simulink model "model_graphicSim_Circuit"  (R2022a)
settings: Solver=FixedStepAuto  StartTime=0.0  StopTime=inf  RelTol=1e-3
values from neighbouring files (symbols this model uses):
  A = 9    [A_circuit_V2_25000.mat]    (also in A_circuit_V2_3167.mat; A_circuit_V3_30000.mat; A_circuit_V3_60000.mat; Configuration.m)
  d = 699840    [A_circuit_V2_25000.mat]    (also in A_circuit_V2_3167.mat; A_circuit_V3_30000.mat; A_circuit_V3_60000.mat; Configuration.m)
  egoID = 1    [A_circuit_V2_25000.mat]    (also in A_circuit_V2_3167.mat; A_circuit_V3_30000.mat; A_circuit_V3_60000.mat; Configuration.m)
  frontDistCG = 3.7    [A_circuit_V2_25000.mat]    (also in A_circuit_V2_3167.mat; A_circuit_V3_30000.mat; A_circuit_V3_60000.mat; Configuration.m)
  gridvx = [-5 -4.72222222222 -4.44444444444 -4.16666666667 -3.88888888889 -3.61111111111 -3.33333333333 -3.05555555556 -2.77777777778 -2.5 0 0.277777777778 ... (70 elements, 10x7)]    [A_circuit_V2_25000.mat]    (also in A_circuit_V2_3167.mat; A_circuit_V3_30000.mat; A_circuit_V3_60000.mat; circuit_10000_P2.mat)
  gridvy = [-70 -68.4444444444 -66.8888888889 -65.3333333333 -63.7777777778 -62.2222222222 -60.6666666667 -59.1111111111 -57.5555555556 -56 -50 -48.4444444444 ... (70 elements, 10x7)]    [A_circuit_V2_25000.mat]    (also in A_circuit_V2_3167.mat; A_circuit_V3_30000.mat; A_circuit_V3_60000.mat; circuit_10000_P2.mat)
  gridx = [-85 -84.6666666667 -84.3333333333 -84 -83.6666666667 -83.3333333333 -83 -82.6666666667 -82.3333333333 -82 -55 -54.6666666667 ... (70 elements, 10x7)]    [A_circuit_V2_25000.mat]    (also in A_circuit_V2_3167.mat; A_circuit_V3_30000.mat; A_circuit_V3_60000.mat; circuit_10000_P2.mat)
  gridy = [-70 -69.3333333333 -68.6666666667 -68 -67.3333333333 -66.6666666667 -66 -65.3333333333 -64.6666666667 -64 -50 -49.3333333333 ... (70 elements, 10x7)]    [A_circuit_V2_25000.mat]    (also in A_circuit_V2_3167.mat; A_circuit_V3_30000.mat; A_circuit_V3_60000.mat; circuit_10000_P2.mat)
  gridyaw = [-504 -489.6 -475.2 -460.8 -446.4 -432 -417.6 -403.2 -388.8 -374.4 -360 -345.6 ... (70 elements, 10x7)]    [A_circuit_V2_25000.mat]    (also in A_circuit_V2_3167.mat; A_circuit_V3_30000.mat; A_circuit_V3_60000.mat; circuit_10000_P2.mat)
  lb_angSt = -1080    [A_circuit_V2_25000.mat]    (also in A_circuit_V2_3167.mat; A_circuit_V3_30000.mat; A_circuit_V3_60000.mat; Configuration.m = -900)
  lbvx = 0    [A_circuit_V2_25000.mat]    (also in A_circuit_V2_3167.mat; A_circuit_V3_30000.mat; A_circuit_V3_60000.mat; Configuration.m = -2)
  lbvy = -50    [A_circuit_V2_25000.mat]    (also in A_circuit_V2_3167.mat; A_circuit_V3_30000.mat; A_circuit_V3_60000.mat; Configuration.m = -20)
  lbx = -55    [A_circuit_V2_25000.mat]    (also in A_circuit_V2_3167.mat; A_circuit_V3_30000.mat; A_circuit_V3_60000.mat; Configuration.m = 0)
  lby = -50    [A_circuit_V2_25000.mat]    (also in A_circuit_V2_3167.mat; A_circuit_V3_30000.mat; A_circuit_V3_60000.mat; Configuration.m = 2)
  leftDistCG = 0.9    [A_circuit_V2_25000.mat]    (also in A_circuit_V2_3167.mat; A_circuit_V3_30000.mat; A_circuit_V3_60000.mat; Configuration.m)
  M = 5    [A_circuit_V2_25000.mat]    (also in A_circuit_V2_3167.mat; A_circuit_V3_30000.mat; A_circuit_V3_60000.mat; Configuration.m)
  N = 10    [A_circuit_V2_25000.mat]    (also in A_circuit_V2_3167.mat; A_circuit_V3_30000.mat; A_circuit_V3_60000.mat; Configuration.m)
  passo_steerang = 45    [A_circuit_V2_25000.mat]    (also in A_circuit_V2_3167.mat; A_circuit_V3_30000.mat; A_circuit_V3_60000.mat; Configuration.m = 180)
  passo_v = 0.5    [A_circuit_V2_25000.mat]    (also in A_circuit_V2_3167.mat; A_circuit_V3_30000.mat; A_circuit_V3_60000.mat; Configuration.m)
  retroDistCG = 1    [A_circuit_V2_25000.mat]    (also in A_circuit_V2_3167.mat; A_circuit_V3_30000.mat; A_circuit_V3_60000.mat; Configuration.m)
  safetyDist = 0.5    [A_circuit_V2_25000.mat]    (also in A_circuit_V2_3167.mat; A_circuit_V3_30000.mat; A_circuit_V3_60000.mat; Configuration.m)
  Ts = 0.1    [A_circuit_V2_25000.mat]    (also in A_circuit_V2_3167.mat; A_circuit_V3_30000.mat; A_circuit_V3_60000.mat; Configuration.m)
  ub_angSt = 1080    [A_circuit_V2_25000.mat]    (also in A_circuit_V2_3167.mat; A_circuit_V3_30000.mat; A_circuit_V3_60000.mat; Configuration.m = 900)
  ubvx = 25    [A_circuit_V2_25000.mat]    (also in A_circuit_V2_3167.mat; A_circuit_V3_30000.mat; A_circuit_V3_60000.mat; Configuration.m = 2)
  ubvy = 50    [A_circuit_V2_25000.mat]    (also in A_circuit_V2_3167.mat; A_circuit_V3_30000.mat; A_circuit_V3_60000.mat; Configuration.m = 20)
  ubx = 95    [A_circuit_V2_25000.mat]    (also in A_circuit_V2_3167.mat; A_circuit_V3_30000.mat; A_circuit_V3_60000.mat; Configuration.m = 25)
  uby = 50    [A_circuit_V2_25000.mat]    (also in A_circuit_V2_3167.mat; A_circuit_V3_30000.mat; A_circuit_V3_60000.mat; Configuration.m = 10)
  w = [0 0 0 0 0 0 0 0 0 0 0 0 ... (699840 elements, 699840x1)]    [A_circuit_V2_25000.mat]    (also in A_circuit_V2_3167.mat; A_circuit_V3_30000.mat; A_circuit_V3_60000.mat; circuit_10000_P2.mat)
  x_0 = 2*rand+19    [Configuration.m]    (also in Configuration_circuit.m = -30; Configuration_circuit_V2.m = 0; Configuration_curve.m = 5; Configuration_curve_2.m = 5)
  y_0 = -(3.5*rand+2)    [Configuration.m]    (also in Configuration_circuit.m = -(-20 - rand*6); Configuration_circuit_V2.m = -(-29.5 - rand*7); Configuration_curve.m = -(1-2.1*rand); Configuration_curve_2.m = -(1-2.1*rand))
  yaw_0 = deg2rad(34)    [Configuration_circuit.m]    (also in Configuration_circuit_V2.m = deg2rad(0); Configuration_curve.m = deg2rad(15); Configuration_curve_2.m = deg2rad(15))
undefined symbols (not defined in the file or in its folder): deg, driving, rad, s
libraries: drivingscenarioandsensors x3, simulink_extras x2, sim3dlib x1, sim3dautolib x1, aerolibconvert2 x1, vehdynlibsteering x1, autolibshared x1
settings Model: Creator=User  LastModifiedBy=User

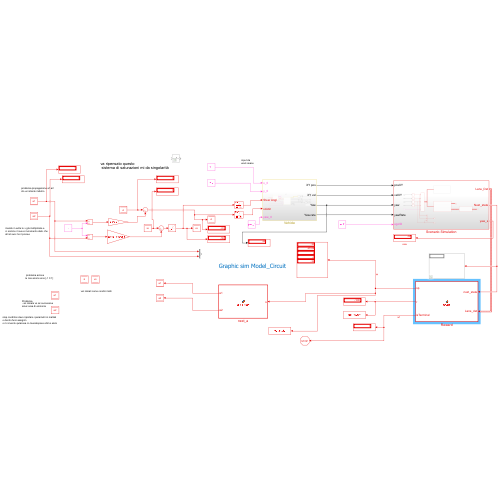
[thumbnail: Simulink's stored preview of the top-level diagram]
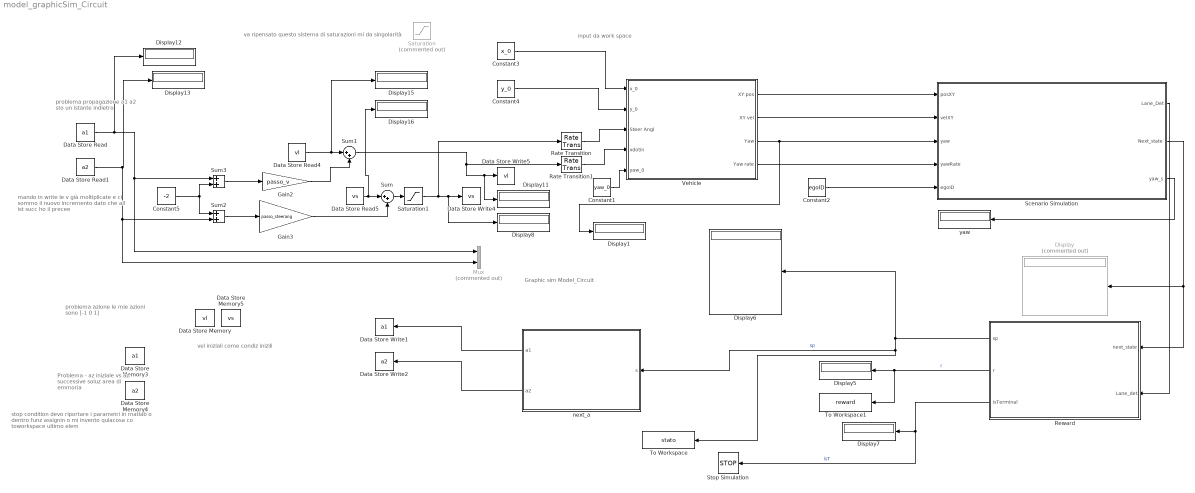
== system model_graphicSim_Circuit ==
  note: va ripensato questo
      | sistema di saturazioni mi da singolarità
  note: mando in write le v già moltiplicate e
      | ci sommo il nuovo incremento dato che
      | all ist succ ho il precee
  note: problema azione
      | le mie azioni sono [-1 0 1]
  note: vel iniziali come condiz inizili
  note: stop condition devo riportare i parametri in matlab
      | o dentro funz assignin
      | o mi invento qulacosa co toworkspace ultimo elem
  note: Problema
      | - az iniziale vs az successive
      | soluz area di emmoria
  note: problema propagazione a1 a2
      | sto un istante indietro
  note: input da work space
  note: Graphic sim Model_Circuit
  Constant1 : Constant  Value=yaw_0
  Constant2 : Constant  Value=egoID
  Constant3 : Constant  Value=x_0
  Constant4 : Constant  Value=y_0
  Constant5 : Constant  Value=-2
  Data Store Memory : DataStoreMemory  DataStoreName=vl  WriteAfterWriteMsg=warning  ShowAdditionalParam=off
  Data Store Memory3 : DataStoreMemory  DataStoreName=a1  WriteAfterWriteMsg=warning  InitialValue=az_1  VectorParams1D=off  ShowAdditionalParam=off  OutDataTypeStr=double
  Data Store Memory4 : DataStoreMemory  DataStoreName=a2  WriteAfterWriteMsg=warning  InitialValue=az_2  VectorParams1D=off  ShowAdditionalParam=off  OutDataTypeStr=double
  Data Store Memory5 : DataStoreMemory  DataStoreName=vs  WriteAfterWriteMsg=warning  ShowAdditionalParam=off
  Data Store Read : DataStoreRead  DataStoreName=a1  IndexOptions=Index vector (dialog)  Indices=1  OutputSizes=1
  Data Store Read1 : DataStoreRead  DataStoreName=a2  IndexOptions=Index vector (dialog)  Indices=1  OutputSizes=1
  Data Store Read4 : DataStoreRead  DataStoreName=vl  IndexOptions=Index vector (dialog)  Indices=1  OutputSizes=1
  Data Store Read5 : DataStoreRead  DataStoreName=vs  IndexOptions=Index vector (dialog)  Indices=1  OutputSizes=1
  Data Store Write1 : DataStoreWrite  DataStoreName=a1  IndexOptions=Index vector (dialog)  Indices=1  OutputSizes=1
  Data Store Write2 : DataStoreWrite  DataStoreName=a2  IndexOptions=Index vector (dialog)  Indices=1  OutputSizes=1
  Data Store Write4 : DataStoreWrite  DataStoreName=vs  IndexOptions=Index vector (dialog)  Indices=1  OutputSizes=1
  Data Store Write5 : DataStoreWrite  DataStoreName=vl  IndexOptions=Index vector (dialog)  Indices=1  OutputSizes=1
  Display : Display  Commented=on
  Display{1,5..8,11..13,15..16} (10 alike) : Display
  Gain2 : Gain  Gain=passo_v
  Gain3 : Gain  Gain=passo_steerang
  Mux : Mux  Commented=on  Inputs=2
  Rate Transition : RateTransition
  Rate Transition1 : RateTransition
  Reward : MATLAB Function  TreatAsAtomicUnit=on
  Saturation : Saturate  Commented=on  UpperLimit=ubvx  LowerLimit=lbvx
  Saturation1 : Saturate  UpperLimit=ub_angSt  LowerLimit=lb_angSt
  Scenario Simulation : Subsystem
  Stop Simulation : Stop
  Sum : Sum  Inputs=|++
  Sum1 : Sum  Inputs=|++
  Sum2 : Sum
  Sum3 : Sum
  To Workspace : ToWorkspace  VariableName=stato  SampleTime=-1
  To Workspace1 : ToWorkspace  VariableName=reward  SampleTime=-1
  Vehicle : Subsystem
  next_a : MATLAB Function  TreatAsAtomicUnit=on
  yaw : Display
  wires:
  Saturation1/1 -> Rate Transition/1, Display8/1, Data Store Write4/1
  Rate Transition/1 -> Vehicle/3(Steer Angl)
  Reward/2(r) -> To Workspace1/1, Display5/1  "r"
  Vehicle/3(Yaw) -> Scenario Simulation/3(yaw), Display1/1
  Gain2/1 -> Sum1/2
  Sum3/1 -> Gain2/1
  Data Store Read5/1 -> Display16/1, Sum/1
  Data Store Read/1 -> Display12/1, Sum3/1, Mux/1
  Sum/1 -> Saturation1/1
  Sum2/1 -> Gain3/1
  Sum1/1 -> Data Store Write5/1, Display11/1, Rate Transition1/1
  Reward/3(isTerminal) -> Stop Simulation/1, Display7/1  "isT"
  Data Store Read1/1 -> Display13/1, Sum2/2, Mux/2
  Constant5/1 -> Sum3/2, Sum2/1
  Gain3/1 -> Sum/2
  Constant3/1 -> Vehicle/1(x_0)
  Data Store Read4/1 -> Display15/1, Sum1/1
  Reward/1(sp) -> Display6/1, To Workspace/1, next_a/1(s)  "sp"
  Vehicle/4(Yaw rate) -> Scenario Simulation/4(yawRate)
  Constant2/1 -> Scenario Simulation/5(egoID)
  Vehicle/2(XY vel) -> Scenario Simulation/2(velXY)
  Rate Transition1/1 -> Vehicle/4(xdotin)
  Vehicle/1(XY pos) -> Scenario Simulation/1(posXY)
  Constant4/1 -> Vehicle/2(y_0)
  next_a/1(a1) -> Data Store Write1/1
  next_a/2(a2) -> Data Store Write2/1
  Constant1/1 -> Vehicle/5(yaw_0)
  Scenario Simulation/2(Next_state) -> Reward/1(next_state), Display/1
  Scenario Simulation/1(Lane_Det) -> Reward/2(Lane_det)
  Scenario Simulation/3(yaw_s) -> yaw/1

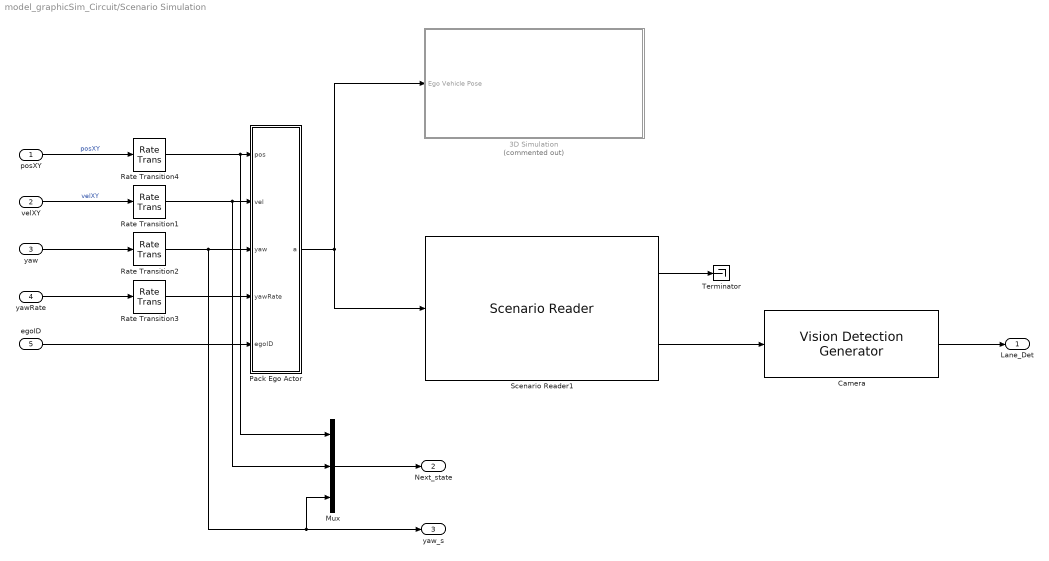
== system model_graphicSim_Circuit/Scenario Simulation ==
  posXY : Inport
  velXY : Inport  Port=2
  yaw : Inport  Port=3
  yawRate : Inport  Port=4
  egoID : Inport  Port=5
  3D Simulation : Subsystem  Commented=on
  Camera : drivingscenarioandsensors/Vision Detection Generator  SensorIndex=1  DetectorOutput=Lanes only  UpdateInterval=0.1  LaneUpdateInterval=0.1  SensorLocation=[0 0]  Height=1.1  Yaw=0  Pitch=1  Roll=0  BusNameSource=Auto  BusName=BusObjectDetections  BusName2Source=Auto  BusName2=BusLaneDetections  MaxNumDetectionsSource=Property  MaxNumDetections=50  MaxNumLanesSource=Property  MaxNumLanes=30  DetectionCoordinates=Ego Cartesian  SimulateUsing=Interpreted execution  MaxRange=150  BoundingBoxAccuracy=5  ProcessNoiseIntensity=5  MaxSpeed=100  MaxAllowedOcclusion=0.5  MinObjectImageSize=[15 15]  DetectionProbability=1  FalsePositivesPerImage=0  MinLaneImageSize=[20 3]  LaneBoundaryAccuracy=3  HasNoise=off  InitialSeedSource=Repeatable  InitialSeed=0  UsedSeed=0  ActorProfilesSource=From Scenario Reader block  ActorProfilesParameters=driving.internal.ActorProfilesParameters  ActorProfilesExpression=[struct('ActorID',1,'ClassID',1,'Length',4.7,'Width',1.8,'Height',1.4,'OriginOffset',[-1.35 0 0],'MeshVertices',[3.7 0.9 0.857439446366782;3.7 -0.9 0.857439446366782;3.7 -0.9 0.314878892733564;3.7 0.9 0.314878892733564;3.7 0.9 0.857439446366782;2.525 0.9 0.993079584775086;2.525 -0.9 0.993079584775086;3.7 -0.9 0.857439446366782;1.82 0.72 1.4;0.41 0.72 1.4;0.41 -0.72 1.4;1.82 -0.72 1.4;-0.295 0.9 0.993079584775086;-1 0.9 0.857439446366782;-1 -0.9 0.857439446366782;-0.295 -0.9 0.993079584775086;3.7 0.9 0.857439446366782;3.7 0.9 0.314878892733564;2.525 0.9 0.314878892733564;2.525 0.9 0.993079584775086;2.525 0.9 0.993079584775086;2.525 0.9 0.314878892733564;-0.295 0.9 0.314878892733564;-0.295 0.9 0.993079584775086;-0.295 0.9 0.993079584775086;-0.295 0.9 0.314878892733564;-1 0.9 0.355570934256055;-1 0.9 0.857439446366782;2.525 0.9 0.993079584775086;-0.295 0.9 0.993079584775086;0.41 0.72 1.4;1.82 0.72 1.4;3.7 -0.9 0.857439446366782;3.7 -0.9 0.314878892733564;2.525 -0.9 0.314878892733564;2.525 -0.9 0.993079584775086;2.525 -0.9 0.993079584775086;2.525 -0.9 0.314878892733564;-0.295 -0.9 0.314878892733564;-0.295 -0.9 0.993079584775086;-0.295 -0.9 0.993079584775086;-0.295 -0.9 0.314878892733564;-1 -0.9 0.355570934256055;-1 -0.9 0.857439446366782;2.525 -0.9 0.993079584775086;-0.295 -0.9 0.993079584775086;0.41 -0.72 1.4;1.82 -0.72 1.4;-0.295 0.9 0.993079584775086;-0.295 -0.9 0.993079584775086;0.41 -0.72 1.4;0.41 0.72 1.4;2.525 -0.9 0.993079584775086;1.82 -0.72 1.4;1.82 0.72 1.4;2.525 0.9 0.993079584775086;-1 0.9 0.857439446366782;-1 0.9 0.355570934256055;-1 -0.9 0.355570934256055;-1 -0.9 0.857439446366782;3.7 0.9 0.314878892733564;3.7 -0.9 0.314878892733564;-0.295 -0.9 0.314878892733564;-0.295 0.9 0.314878892733564;-0.295 0.9 0.314878892733564;-1 0.9 0.355570934256055;-1 -0.9 0.355570934256055;-0.295 -0.9 0.314878892733564;0 -0.63 0;0 -0.87 0;0.191030206995054 -0.63 0.0601365173421445;0.191030206995054 -0.87 0.0601365173421445;0.309093367795925 -0.63 0.217575963708927;0.309093367795925 -0.87 0.217575963708927;0.309093367795925 -0.63 0.412181821758201;0.309093367795925 -0.87 0.412181821758201;0.191030206995054 -0.63 0.569621268124983;0.191030206995054 -0.87 0.569621268124983;0 -0.63 0.629757785467128;0 -0.87 0.629757785467128;-0.191030206995054 -0.63 0.569621268124983;-0.191030206995054 -0.87 0.569621268124983;-0.309093367795925 -0.63 0.412181821758201;-0.309093367795925 -0.87 0.412181821758201;-0.309093367795925 -0.63 0.217575963708927;-0.309093367795925 -0.87 0.217575963708927;-0.191030206995054 -0.63 0.0601365173421445;-0.191030206995054 -0.87 0.0601365173421445;0 -0.63 0;0 -0.87 0;0 -0.63 0;0.191030206995054 -0.63 0.0601365173421445;0.309093367795925 -0.63 0.217575963708927;0.309093367795925 -0.63 0.412181821758201;0.191030206995054 -0.63 0.569621268124983;0 -0.63 0.629757785467128;-0.191030206995054 -0.63 0.569621268124983;-0.309093367795925 -0.63 0.412181821758201;-0.309093367795925 -0.63 0.217575963708927;-0.191030206995054 -0.63 0.0601365173421445;0 -0.87 0;0.191030206995054 -0.87 0.0601365173421445;0.309093367795925 -0.87 0.217575963708927;0.309093367795925 -0.87 0.412181821758201;0.191030206995054 -0.87 0.569621268124983;0 -0.87 0.629757785467128;-0.191030206995054 -0.87 0.569621268124983;-0.309093367795925 -0.87 0.412181821758201;-0.309093367795925 -0.87 0.217575963708927;-0.191030206995054 -0.87 0.0601365173421445;0 0.87 0;0 0.63 0;0.191030206995054 0.87 0.0601365173421445;0.191030206995054 0.63 0.0601365173421445;0.309093367795925 0.87 0.217575963708927;0.309093367795925 0.63 0.217575963708927;0.309093367795925 0.87 0.412181821758201;0.309093367795925 0.63 0.412181821758201;0.191030206995054 0.87 0.569621268124983;0.191030206995054 0.63 0.569621268124983;0 0.87 0.629757785467128;0 0.63 0.629757785467128;-0.191030206995054 0.87 0.569621268124983;-0.191030206995054 0.63 0.569621268124983;-0.309093367795925 0.87 0.412181821758201;-0.309093367795925 0.63 0.412181821758201;-0.309093367795925 0.87 0.217575963708927;-0.309093367795925 0.63 0.217575963708927;-0.191030206995054 0.87 0.0601365173421445;-0.191030206995054 0.63 0.0601365173421445;0 ...(+3718 chars)],'MeshFaces',[1 2 3;3 4 1;5 6 7;7 8 5;9 10 11;11 12 9;13 14 15;15 16 13;17 18 19;19 20 17;21 22 23;23 24 21;25 26 27;27 28 25;29 30 31;31 32 29;33 34 35;35 36 33;37 38 39;39 40 37;41 42 43;43 44 41;45 46 47;47 48 45;49 50 51;51 52 49;53 54 55;55 56 53;57 58 59;59 60 57;61 62 63;63 64 61;65 66 67;67 68 65;69 71 72;72 70 69;71 73 74;74 72 71;73 75 76;76 74 73;75 77 78;78 76 75;77 79 80;80 78 77;79 81 82;82 80 79;81 83 84;84 82 81;83 85 86;86 84 83;85 87 88;88 86 85;87 89 90;90 88 87;91 92 93;91 93 94;91 94 95;91 95 96;91 96 97;91 97 98;91 98 99;91 99 100;101 102 103;101 103 104;101 104 105;101 105 106;101 106 107;101 107 108;101 108 109;101 109 110;111 113 114;114 112 111;113 115 116;116 114 113;115 117 118;118 116 115;117 119 120;120 118 117;119 121 122;122 120 119;121 123 124;124 122 121;123 125 126;126 124 123;125 127 128;128 126 125;127 129 130;130 128 127;129 131 132;132 130 129;133 134 135;133 135 136;133 136 137;133 137 138;133 138 139;133 139 140;133 140 141;133 141 142;143 144 145;143 145 146;143 146 147;143 147 148;143 148 149;143 149 150;143 150 151;143 151 152;153 155 156;156 154 153;155 157 158;158 156 155;157 159 160;160 158 157;159 161 162;162 160 159;161 163 164;164 162 161;163 165 166;166 164 163;165 167 168;168 166 165;167 169 170;170 168 167;169 171 172;172 170 169;171 173 174;174 172 171;175 176 177;175 177 178;175 178 179;175 179 180;175 180 181;175 181 182;175 182 183;175 183 184;185 186 187;185 187 188;185 188 189;185 189 190;185 190 191;185 191 192;185 192 193;185 193 194;195 197 198;198 196 195;197 199 200;200 198 197;199 201 202;202 200 199;201 203 204;204 202 201;203 205 206;206 204 203;205 207 208;208 206 205;207 209 210;210 208 207;209 211 212;212 210 209;211 213 214;214 212 211;213 215 216;216 214 213;217 218 219;217 219 220;217 220 221;217 221 222;217 222 223;217 223 224;217 224 225;217 225 226;227 228 229;227 229 230;227 230 231;227 231 232;227 232 233;227 233 234;227 234 235;227 235 236],'RCSPattern',[10 10;10 10],'RCSAzimuthAngles',[-180 180],'RCSElevationAngles',[-90 90])]  Intrinsics=driving.internal.cameraIntrinsics('FocalLength',[300 800],'PrincipalPoint',[320 240],'ImageSize',[480 640],'RadialDistortion',[0 0],'TangentialDistortion',[0 0],'Skew',0)
  Mux : Mux  Inputs=3
  Pack Ego Actor : MATLAB Function  TreatAsAtomicUnit=on
  Rate Transition{1..4} (4 alike) : RateTransition  OutPortSampleTime=Ts
  Scenario Reader1 : drivingscenarioandsensors/Scenario Reader  ScenarioSource=From file  ScenarioFileName=C:\Users\User\OneDrive\Desktop\ThesisProject\project\scenario_circuit.mat  ScenarioVariableName=scenario  OutputCoordinateSystem=Vehicle coordinates  EgoVehicleSource=Input port  EgoVehicleActorID=1  OrientVehiclesOnRoad=off  OutputEgoVehiclePose=off  OutputEgoVehicleState=off  SampleTime=Ts  LaneBoundaryOutput=Ego vehicle lane boundaries  LaneBoundaryDistance=linspace(-150, 150, 101)  LaneBoundaryLocation=Center of lane markings  BusNameSource=Auto  BusName=BusActors  BusNumActorsSource=Scenario  BusNumActors=100  BusName2Source=Auto  BusName2=BusLaneBoundaries  BusNumLaneBoundariesSource=Scenario  BusNumLaneBoundaries=10  BusName3Source=Auto  BusName3=BusEgoActor  BusName4Source=Auto  BusName4=BusEgoState  ShowCoordinateLabels=on  SimulateUsing=Interpreted execution
  Terminator : Terminator
  Lane_Det : Outport
  Next_state : Outport  Port=2
  yaw_s : Outport  Port=3
  wires:
  Pack Ego Actor/1(a) -> Scenario Reader1/1, 3D Simulation/1(Ego Vehicle Pose)
  yawRate/1 -> Rate Transition3/1
  Rate Transition1/1 -> Mux/2, Pack Ego Actor/2(vel)
  Rate Transition4/1 -> Mux/1, Pack Ego Actor/1(pos)
  Rate Transition3/1 -> Pack Ego Actor/4(yawRate)
  Rate Transition2/1 -> Mux/3, yaw_s/1, Pack Ego Actor/3(yaw)
  egoID/1 -> Pack Ego Actor/5(egoID)
  velXY/1 -> Rate Transition1/1  "velXY"
  posXY/1 -> Rate Transition4/1  "posXY"
  yaw/1 -> Rate Transition2/1
  Mux/1 -> Next_state/1
  Scenario Reader1/1 -> Terminator/1
  Camera/1 -> Lane_Det/1
  Scenario Reader1/2 -> Camera/1

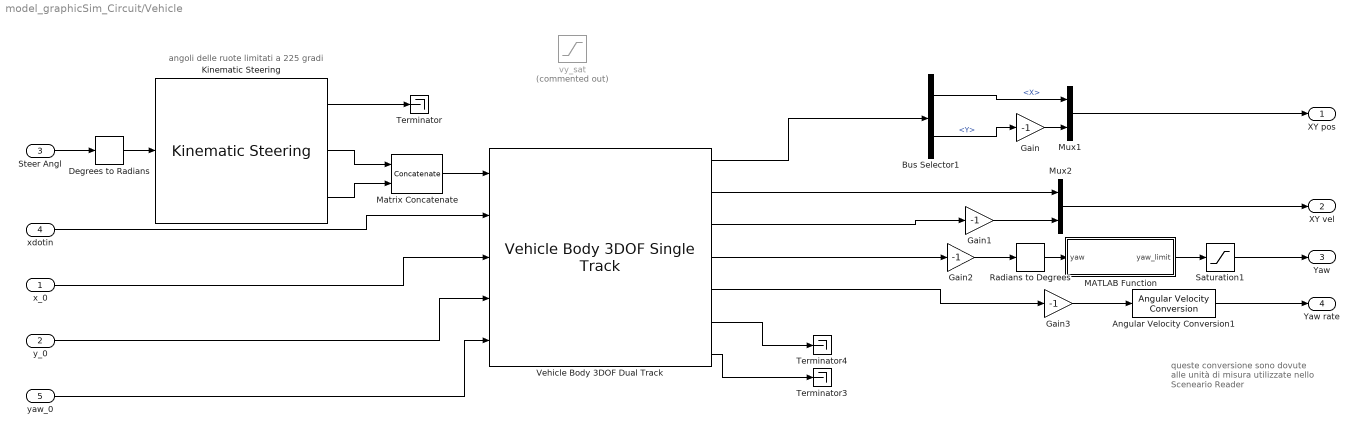
== system model_graphicSim_Circuit/Vehicle ==
  note: angoli delle ruote limitati a 225 gradi
  note: queste conversione sono dovute
      | alle unità di misura utilizzate nello
      | Sceneario Reader
  x_0 : Inport
  y_0 : Inport  Port=2
  Steer Angl : Inport  Port=3
  xdotin : Inport  Port=4
  yaw_0 : Inport  Port=5
  Angular Velocity Conversion1 : aerolibconvert2/Angular Velocity Conversion  IU=rad/s  OU=deg/s
  Bus Selector1 : BusSelector  OutputSignals=InertFrm.Cg.Disp.X,InertFrm.Cg.Disp.Y
  Degrees to Radians : simulink_extras/Transformations/Degrees to Radians
  Gain{,1..3} (4 alike) : Gain  Gain=-1
  Kinematic Steering : vehdynlibsteering/Kinematic Steering  StrgType=Ackerman  StrgRatioType=Constant  Loc=Front  NrmlFctr=0.01  TrckWdth=1  WhlBase=1.524  Db=0  StrgRng=9*pi  StrgAngBpts="[-6.2832   -5.0265   -3.7699   -2.5133   -1.2566         0    1.2566    2.5133    3.7699    5.0265    6.2832]"  StrgRatioTbl=|  StrgRatio=100  PctAckIn=off  PctAck=100  PctAckTbl=ones(1,11)*100  StrgArmLngth=0.1  RckCsLngth=0.5  TieRodLngth=0.248  D=0.2  PnnRadius=0.00085818  PnnRadiusTbl="[0.0055    0.0055    0.0056    0.0057    0.0058    0.0057    0.0057    0.0057    0.0056    0.0055    0.0055]"  RodLngth=0.1  ParaArmLngth=0.9  aMode=2
      | [13.5000   13.3750   13.2500   13.1250   13.0000   13.0000   13.0000   13.1250   13.2500   13.3750   13.5000
      | ]
  MATLAB Function : MATLAB Function  TreatAsAtomicUnit=on
  Matrix Concatenate : Concatenate  ConcatenateDimension=2
  Mux1 : Mux  Inputs=2
  Mux2 : Mux  Inputs=2
  Radians to Degrees : simulink_extras/Transformations/Radians to Degrees
  Saturation1 : Saturate  UpperLimit=360  LowerLimit=-360
  Terminator : Terminator
  Terminator3 : Terminator
  Terminator4 : Terminator
  Vehicle Body 3DOF Dual Track : autolibshared/Vehicle Body 3DOF Single Track  trackMode=Dual  inputMode=External longitudinal velocity  frontSteerMode=on  rearSteerMode=off  windMode=off  muMode=off  extFMode=off  extMMode=off  htchFMode=off  htchMMode=off  extXo=on  extpsio=on  extxdoto=off  extro=off  extYo=on  extTamb=off  extydoto=off  aMode=2  NF=2  NR=2  m=2000  a=1.4  b=1.6  h=0.35  dh=1  hh=0.2  X_o=0  xdot_o=0  CalphaMode=off  sigmaMode=on  d=0  hl=0  w=[1.4,1.4]  Cy_f=12e3  Cy_r=11e3  sigma_f=.1  sigma_r=.1  alpha_f_brk=[-.1 .1]  Cy_f_data=[-9e3 9e3]  alpha_r_brk=[-.1 .1]  Cy_r_data=[-9e3 9e3]  Y_o=0  ydot_o=0  Izz=4000  psi_o=0  r_o=0  Af=2  Cd=.3  Cl=.1  Cpm=.1  beta_w=[0 0.01:0.01:0.3]  Cs=[0:0.03:0.9]  Cym=[0 1e-6:0.01:0.3]  Pabs=101325  Tair=273  g=9.81  mu=1  xdot_tol=.01  Fznom=5000  Fxtire_sat=7e4  Fytire_sat=7e4  longOff=0  latOff=0  vertOff=0  wrapAng=off
      settings: SourceProductBaseCode=PW,DR,MT,VE
  vy_sat : Saturate  Commented=on  UpperLimit=ubvy  LowerLimit=lbvy
  XY pos : Outport
  XY vel : Outport  Port=2
  Yaw : Outport  Port=3
  Yaw rate : Outport  Port=4
  wires:
  Bus Selector1/2 -> Gain/1  "<Y>"
  Kinematic Steering/3 -> Matrix Concatenate/2
  Matrix Concatenate/1 -> Vehicle Body 3DOF Dual Track/1
  Vehicle Body 3DOF Dual Track/6 -> Terminator4/1
  Mux1/1 -> XY pos/1
  Bus Selector1/1 -> Mux1/1  "<X>"
  Kinematic Steering/1 -> Terminator/1
  Degrees to Radians/1 -> Kinematic Steering/1
  Vehicle Body 3DOF Dual Track/7 -> Terminator3/1
  Kinematic Steering/2 -> Matrix Concatenate/1
  Mux2/1 -> XY vel/1
  Steer Angl/1 -> Degrees to Radians/1
  xdotin/1 -> Vehicle Body 3DOF Dual Track/2
  Radians to Degrees/1 -> MATLAB Function/1(yaw)
  Gain3/1 -> Angular Velocity Conversion1/1
  x_0/1 -> Vehicle Body 3DOF Dual Track/3
  y_0/1 -> Vehicle Body 3DOF Dual Track/4
  Vehicle Body 3DOF Dual Track/3 -> Gain1/1
  MATLAB Function/1(yaw_limit) -> Saturation1/1
  Saturation1/1 -> Yaw/1
  Vehicle Body 3DOF Dual Track/2 -> Mux2/1
  Vehicle Body 3DOF Dual Track/1 -> Bus Selector1/1
  Gain/1 -> Mux1/2
  Gain1/1 -> Mux2/2
  Gain2/1 -> Radians to Degrees/1
  Vehicle Body 3DOF Dual Track/5 -> Gain3/1
  Vehicle Body 3DOF Dual Track/4 -> Gain2/1
  Angular Velocity Conversion1/1 -> Yaw rate/1
  yaw_0/1 -> Vehicle Body 3DOF Dual Track/5

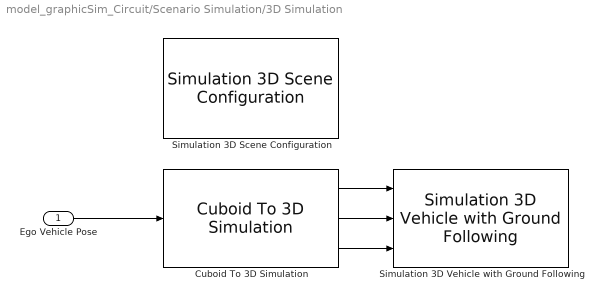
== system model_graphicSim_Circuit/Scenario Simulation/3D Simulation ==
  Ego Vehicle Pose : Inport
  Cuboid To 3D Simulation : drivingscenarioandsensors/Cuboid To 3D Simulation  SpecifyActorID=on  ActorIDToConvert=1  SimulateUsing=Interpreted execution
      settings: SourceProductBaseCode=DR
  Simulation 3D Scene Configuration : sim3dlib/Simulation 3D Scene Configuration  Priority=0  ProjectFormat=Default Scenes  SceneDesc=Straight road  ProjectName=C:\Program Files\MATLAB\R2022a\toolbox\shared\sim3d_projects\automotive_project\UE4\WindowsNoEditor\VehicleSimulation.exe  ScenePath=/Game/Maps/HwStrght  vehTagList={'Scene Origin';'SimulinkVehicle1'}  vehTag=SimulinkVehicle1  OpVisEn=off  Ts=1/60  EnableWindow=on  EnableRemoteAccess=off  EnableWeather=off  SunAltitude=40.0  SunAzimuth=90  clouds=10  wind=1  fog=0  rain=0  sensorTag=MainCamera1  sensorId=1  sensorName=MainCamera1  mountLoc=Origin  offsetFlag=off  tmountOffset=[0, 0, 0]  rmountOffset=[0, 0, 0]  HorizontalResolution=1280  VerticalResolution=720  HorizontalFOV=60  mountPoint=[0 0 0]  mountOrientation=[0 0 0]  aMode=3  ID=1
      settings: SourceProductBaseCode=VE,AE,DR,UV,VE
  Simulation 3D Vehicle with Ground Following : sim3dautolib/Simulation 3D Vehicle with Ground Following  Priority=-1  PassVehMesh=Muscle car  MeshPath=/MathWorksSimulation/Vehicles/Muscle/Meshes/SK_MuscleCar.SK_MuscleCar  TrackWidth=1.9  WheelBase=3  WheelRadius=0.35  VehColor=Red  InitialPos=[0, 0, 0]  InitialRot=[0, 0, 0]  ActorName=SimulinkVehicle1  SampleTime=-1  ActorType=SimulinkVehicle  ID=1  aMode=3  ActorTag=SimulinkVehicle1  CoordinateScheme=ISO  VehLightsControl=off  HeadlightColor=[ 1, 1, 1 ]  HighBeamIntensity=100000  LowBeamIntensity=60000  HighBeamConeAngle=70  LowBeamConeAngle=70  LeftHeadlightOrientation=[ 0, 0 ]  RightHeadlightOrientation=[ 0, 0 ]  BrakelightIntensity=500  ReverselightIntensity=500  SignallightIntensity=500  SignallightPeriod=1  SignalPulseWidth=50  TransformOutportEnabled=off
      settings: SourceProductBaseCode=VE,AE,DR,UV,VE
  wires:
  Cuboid To 3D Simulation/3 -> Simulation 3D Vehicle with Ground Following/3
  Cuboid To 3D Simulation/2 -> Simulation 3D Vehicle with Ground Following/2
  Cuboid To 3D Simulation/1 -> Simulation 3D Vehicle with Ground Following/1
  Ego Vehicle Pose/1 -> Cuboid To 3D Simulation/1

== matlab function model_graphicSim_Circuit/next_a ==
  data: s input; a1 output; gridx parameter; gridy parameter; gridvx parameter; gridvy parameter; gridyaw parameter; M parameter; N parameter; A parameter; d parameter; eps parameter; w parameter; a2 output
function [a1,a2] = eps_greedy(s, gridx, gridy, gridvx, gridvy, gridyaw, M, N, A, d, eps, w)

%s(5) = -s(5);

if rand < eps   % azione random
    a = randi(A); % da 1 a 9 se uso indice
else
    q = zeros(A, 1);
    for a = 1:A  % valuto tutte le azioni che posso prendere
        q(a) = w'*get_features(s, a, gridx, gridy, gridvx, gridvy, gridyaw, M, N, A, d); % approsimazione della funz qualità
    end        % pesi per vett features
    a = find(q == max(q), 1, 'first'); % scelgo quella con funz qualità massima
end

[b1,b2] = ind2sub([3 3],a);

% [1 2 3] vanno mappati su -1,0, con (-2)

if(b1 == 1)
    a1 = 1;
elseif(b1 == 2)
    a1 = 2;
else
    a1 = 3;
end

if(b2 == 1)
    a2 = 1;
elseif(b2 == 2)
    a2 = 2;
else
    a2 = 3;
end

end


function x = get_features(s, a, gridx, gridy, gridvx, gridvy, gridyaw, M, N, A, d)

%coder.extrinsic('assignin')

% numero celle, +1 perchè ne ho aggiunta una
%nCells = (M + 1)^4; % dimensione features per una cella
%d = A*N*nCells; % dimensione vettore pesi da aggiornare
x = zeros(d, 1);
% va modificaro sta dimension var
for ii = 1 : N
    xxx = gridx(ii, :);
    yyy = gridy(ii, :);
    vxvxvx = gridvx(ii, :);
    vyvyvy = gridvy(ii, :);
    yawyawyaw = gridyaw(ii, :);
    % capire in quale cella mi trovo, trovo indice lungo x e lungo y
    ix = find(s(1) >= xxx(1:end-1) & s(1) <= xxx(2:end), 1, 'first');
    iy = find(s(2) >= yyy(1:end-1) & s(2) <= yyy(2:end), 1, 'first');
    ivx = find(s(3) >= vxvxvx(1:end-1) & s(3) <= vxvxvx(2:end), 1, 'first');
    ivy = find(s(4) >= vyvyvy(1:end-1) & s(4) <= vyvyvy(2:end), 1, 'first');
    iyaw = find(s(5) >= yawyawyaw(1:end-1) & s(5) <= yawyawyaw(2:end), 1, 'first');

    % a_ind = sub2ind([3 3],a(1),a(2)); non serve gli passo indice poi da
    % indice a azione quando la uso in dinamica
    % dato doppia dim dell'azione devo subind anche a ???

    % debug
    %pippo = struct('ix',{ix},'iy', {iy},'ivx', {ivx},'ivy', {ivy},'ii', {ii},'a', {a},'s', {s});
    %assignin("base","pippo",pippo);
    % ind = sub2ind([M + 1, M + 1, M + 1, M + 1, N, A], ix, iy, ivx, ivy, ii, a);
    ind = sub2ind([M + 1, M + 1, M + 1, M + 1, M + 1, N, A], ix, iy, ivx, ivy, iyaw, ii, a);

    x(ind) = 1; % valore corrispondente alla cella
    % vett features ha un 1 per ogni griglia
end
end

== matlab function model_graphicSim_Circuit/Reward ==
  data: sp output; next_state input; Lane_det input; r output; isTerminal output; safetyDist parameter; leftDistCG parameter; frontDistCG parameter; retroDistCG parameter; ubx parameter; lbx parameter; uby parameter; lby parameter; lbvx parameter; ubvx parameter
function [sp , r, isTerminal] = reward(next_state, Lane_det, safetyDist, leftDistCG, frontDistCG, retroDistCG,ubx, lbx, uby, lby,lbvx, ubvx)
% CG centro asse posteriore

sp = next_state;

%fatti cosi sto considerando il centro ma la mia macchina ha delle dimensioni e anche orientamento yaw
% se considero misure CG alla fine sto considerando spazio più grande
if((next_state(1) < lbx) )
    sp(1) = lbx;
    r = -1000;
    isTerminal = 1;
    return
elseif(next_state(1) > ubx)
    sp(1) = ubx;
    r = -1000;               
    isTerminal = 1;
    return
elseif(next_state(2) < lby)
    sp(2) = lby;
    r = -1000;              
    isTerminal = 1;
    return
elseif(next_state(2) > uby)
    sp(2) = uby;
    r = -1000;
    isTerminal = 1;
    return
end

if(sp(3) < lbvx) 
    sp(3) = lbvx;
    r = -1000;
    isTerminal = 1;
    return
elseif(sp(3) > ubvx)
    sp(3) = ubvx;
     r = -1000;
    isTerminal = 1;
    return
end

% 
% %LEFT CRASH
% i = 1;
% while(RadSx.Detections(i).Measurement(2) ~= 0) % posizione ritornata va triangolata ???
%     % Front controllo su x
%     if((abs(RadSx.Detections(i).Measurement(2)) - leftDistCG) < safetyDist)
%         r = -1000;
%         isTerminal = 1;
%         return
%     end
%     i = i + 1;
% end
% 
% %RIGHT CRASH
% i = 1;
% while(RadDx.Detections(i).Measurement(2) ~= 0) % posizione ritornata va triangolata ???
%     % Front controllo su x
%     if((abs(RadDx.Detections(i).Measurement(2)) - leftDistCG) < safetyDist)
%         r = -1000;
%         isTerminal = 1;
%         return
%     end
%     i = i + 1;
% end

% CONTROLLO NO LANE DETECTION
if((isnan(Lane_det.LaneBoundaries(1).LateralOffset)) && (isnan(Lane_det.LaneBoundaries(2).LateralOffset)))
    %y = Lane_det.LaneBoundaries(1).LateralOffset;  % possibiltà nan
    %y = Lane_det.LaneBoundaries(2).LateralOffset;

    r = -1000;
    isTerminal = 1;
    return
end

% if((abs(Lane_det.LaneBoundaries(1).LateralOffset)) < leftDistCG+0.1 || abs(Lane_det.LaneBoundaries(2).LateralOffset) < leftDistCG+0.1)
% 
%     r = -1000;
%     isTerminal = 1;
%     return
% end


% CONTROLLO STATO TERMINALE se buco il traguardo
% controllo se sto nella zona terminale

%if((sp(1) >= 10 && sp(1) <= 20)  && (sp(2) >= -38.8 && sp(2) <= -28.8))
%if((sp(1) >= 40)&& (sp(2)<=-28 && sp(2)>=-36))
if((sp(1) >= 10))
    r = 0;
    isTerminal = 1;
    return
end

r = -1;
isTerminal = 0;

== matlab function model_graphicSim_Circuit/Vehicle/MATLAB Function ==
  data: yaw input; yaw_limit output
function yaw_limit = fcn(yaw)

if(yaw > 360)
    yaw_limit = yaw - 360;

elseif(yaw < -360)
     yaw_limit = yaw + 360;
else
    yaw_limit = yaw;
end

end

== matlab function model_graphicSim_Circuit/Scenario Simulation/Pack Ego Actor ==
  data: pos input; a output Bus: BusActors1Actors size=1; vel input; yaw input; yawRate input; egoID input
function a = packEgo(pos,vel,yaw,yawRate,egoID)
% Pack ego information into a single ego actor bus
%
% Imoprtant note:
% Output is a bus of type BusActorsActors. This is the same bus used by the
% Scenario Reader to output an individual actor. If you change the
% output bus name of Scenario Reader change the output bus name here
% as well by clicking on 'Edit Data' in the menu above.

a = struct(...
    'ActorID',egoID,...
    'Position', [pos(1) pos(2) 0], ...
    'Velocity', [vel(1) vel(2) 0], ...
    'Roll', 0, ...
    'Pitch', 0, ...
    'Yaw', yaw, ...
    'AngularVelocity', [0 0 yawRate]);
